simulink model "eqtn2"  (R2017a)
settings: Solver=VariableStepAuto  StartTime=0.0  StopTime=10.0  RelTol=1e-3
settings Model: Creator=misbah  LastModifiedBy=misbah

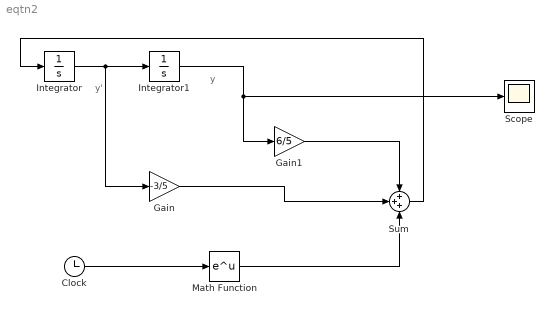
== system eqtn2 ==
  note: y
  note: y'
  Clock : Clock
  Gain : Gain  Gain=-3/5
  Gain1 : Gain  Gain=6/5
  Integrator : Integrator
  Integrator1 : Integrator
  Math Function : Math  SaturateOnIntegerOverflow=on
  Scope : Scope
  Sum : Sum  Inputs=+++
  wires:
  Integrator/1 -> Gain/1, Integrator1/1
  Integrator1/1 -> Scope/1, Gain1/1
  Clock/1 -> Math Function/1
  Gain1/1 -> Sum/1
  Gain/1 -> Sum/2
  Math Function/1 -> Sum/3
  Sum/1 -> Integrator/1
